simulink model "Ackermannsteering"  (R2024b)
settings: Solver=VariableStepAuto  StartTime=0.0  StopTime=10.0  RelTol=1e-3
settings Model: Creator=rober  LastModifiedBy=rober

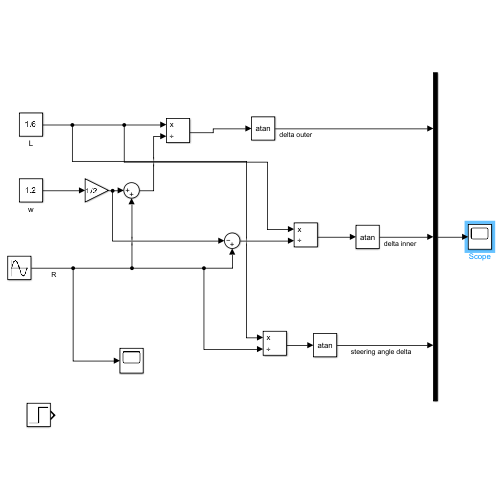
[thumbnail: Simulink's stored preview of the top-level diagram]
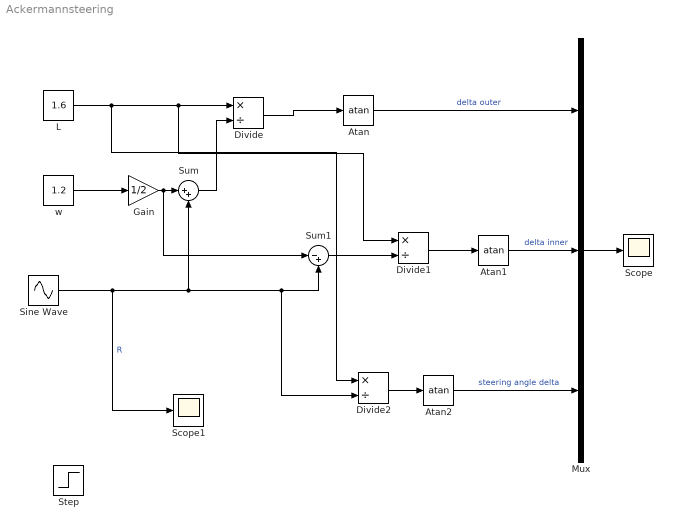
== system Ackermannsteering ==
  Atan : Trigonometry  Operator=atan
  Atan1 : Trigonometry  Operator=atan
  Atan2 : Trigonometry  Operator=atan
  Divide : Product  Inputs=*/
  Divide1 : Product  Inputs=*/
  Divide2 : Product  Inputs=*/
  Gain : Gain  Gain=1/2
  L : Constant  Value=1.6
  Mux : Mux  Inputs=3
  Scope : Scope
  Scope1 : Scope
  Sine Wave : Sin  Amplitude=2  Frequency=0.5  Phase=4  SampleTime=0
  Step : Step  SampleTime=0
  Sum : Sum  Inputs=|++
  Sum1 : Sum  Inputs=|-+
  w : Constant  Value=1.2
  wires:
  w/1 -> Gain/1
  Sine Wave/1 -> Scope1/1, Divide2/2, Sum1/2, Sum/2  "R"
  Gain/1 -> Sum1/1, Sum/1
  Sum/1 -> Divide/2
  L/1 -> Divide2/1, Divide1/1, Divide/1
  Divide/1 -> Atan/1
  Sum1/1 -> Divide1/2
  Divide1/1 -> Atan1/1
  Atan/1 -> Mux/1  "delta outer"
  Mux/1 -> Scope/1
  Divide2/1 -> Atan2/1
  Atan2/1 -> Mux/3  "steering angle delta"
  Atan1/1 -> Mux/2  "delta inner"
